simulink model "Simulink Model"  (R2020b)
settings: Solver=VariableStepAuto  StartTime=0.0  StopTime=10  RelTol=1e-3
undefined symbols (not defined in the file): a1, a2, g, R, r, v1, v2, v3, w, x, y, z
libraries: simulink_extras x1
settings Model: Creator=Dow69  LastModifiedBy=Dow69

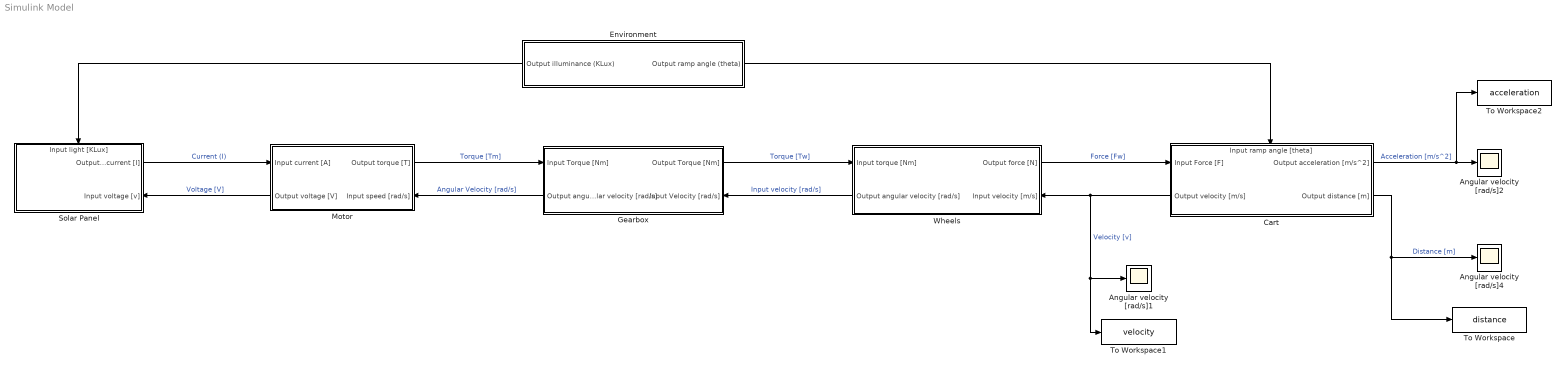
== system Simulink Model ==
  Angular velocity [rad/s]1 : Scope
  Angular velocity [rad/s]2 : Scope
  Angular velocity [rad/s]4 : Scope
  Cart : Subsystem  mask{m=1.319}
      mask prompts: m "Enter cart mass in kg"
      settings: PortSchema="{\"entries\":[{\"content\":{\"sides\":[{\"content\":{\"connectorIds\":[\"In1\",\"Out3\"]},\"type\":\"ConnectorPlacement.EquallySpacedRectSide\",\"uuid\":\"405a4784-f51f-4905-a480-0161a7144eef\"},{\"content\":{\"connectorIds\":[\"Out1\",\"Out2\"],\"side\":\"RIGHT\"},\"type\":\"ConnectorPlacement.EquallySpacedRectSide\",\"uuid\":\"ea7e0711-03fc-41b1-ba47-98d5601a56bc\"},{\"content\":{\"connectorIds\":[\"In2\"],\"side\":\"TOP\"},\"type\":\"ConnectorPlacement.EquallySpacedRectSide\",\"uuid\":\"329a5e39-ca06-4825-98ae-3bcb1db21222\"},{\"content\":{\"connectorIds\":[],\"side\":\"HIDDEN\"},\"type\":\"ConnectorPlacement.EquallySpacedRectSide\",\"uuid\":\"bdc78aba-688e-4dc2-92c3-421802cb88ce\"}]},\"type\":\"ConnectorPlacement.EquallySpacedConnector\",\"uuid\":\"ce64d1b9-0ca5-491b-8110-30a1d080445d\"}],\"packageUris\":[\"http://schema.mathworks.com/mf0/Connector/R2020b\"],\"version\":\"1.0\"}"
  Environment : Subsystem  mask{L=20, a=6.1}
      mask prompts: L "Enter illuminance in KLux"; a "Enter angle in degrees"
      settings: PortSchema="{\"entries\":[{\"content\":{\"sides\":[{\"content\":{\"connectorIds\":[\"Out2\"]},\"type\":\"ConnectorPlacement.EquallySpacedRectSide\",\"uuid\":\"216ba352-b268-472c-abbe-3cb1921569eb\"},{\"content\":{\"connectorIds\":[\"Out1\"],\"side\":\"RIGHT\"},\"type\":\"ConnectorPlacement.EquallySpacedRectSide\",\"uuid\":\"9aa5a236-758d-475f-983b-3b65685f354e\"},{\"content\":{\"connectorIds\":[],\"side\":\"TOP\"},\"type\":\"ConnectorPlacement.EquallySpacedRectSide\",\"uuid\":\"b54bcaaf-885b-4bc1-bf6d-84ce1f01bed9\"},{\"content\":{\"connectorIds\":[],\"side\":\"HIDDEN\"},\"type\":\"ConnectorPlacement.EquallySpacedRectSide\",\"uuid\":\"dd7d4bf7-52e6-41b8-b6d7-f11b8ad94410\"}]},\"type\":\"ConnectorPlacement.EquallySpacedConnector\",\"uuid\":\"024e2dd2-e0e3-4e08-8446-8a7f5dd20cd0\"}],\"packageUris\":[\"http://schema.mathworks.com/mf0/Connector/R2020b\"],\"version\":\"1.0\"}"
  Gearbox : Subsystem
      settings: PortSchema="{\"entries\":[{\"content\":{\"sides\":[{\"content\":{\"connectorIds\":[\"In1\",\"Out2\"]},\"type\":\"ConnectorPlacement.EquallySpacedRectSide\",\"uuid\":\"8709382a-be33-43d3-8815-e6eab9f7b0e2\"},{\"content\":{\"connectorIds\":[\"Out1\",\"In2\"],\"side\":\"RIGHT\"},\"type\":\"ConnectorPlacement.EquallySpacedRectSide\",\"uuid\":\"0ff964dc-029b-47ae-a4ba-260b3c732ea2\"},{\"content\":{\"connectorIds\":[],\"side\":\"TOP\"},\"type\":\"ConnectorPlacement.EquallySpacedRectSide\",\"uuid\":\"270be714-ac21-48e6-9a25-87552b992944\"},{\"content\":{\"connectorIds\":[],\"side\":\"HIDDEN\"},\"type\":\"ConnectorPlacement.EquallySpacedRectSide\",\"uuid\":\"9bfe0afb-4326-44a4-9bc7-f5e5f9747662\"}]},\"type\":\"ConnectorPlacement.EquallySpacedConnector\",\"uuid\":\"0c65735c-987a-4693-bab6-a5fdb23f2f10\"}],\"packageUris\":[\"http://schema.mathworks.com/mf0/Connector/R2020b\"],\"version\":\"1.0\"}"
  Motor : Subsystem
      settings: PortSchema="{\"entries\":[{\"content\":{\"sides\":[{\"content\":{\"connectorIds\":[\"In1\",\"Out2\"]},\"type\":\"ConnectorPlacement.EquallySpacedRectSide\",\"uuid\":\"8709382a-be33-43d3-8815-e6eab9f7b0e2\"},{\"content\":{\"connectorIds\":[\"Out1\",\"In2\"],\"side\":\"RIGHT\"},\"type\":\"ConnectorPlacement.EquallySpacedRectSide\",\"uuid\":\"0ff964dc-029b-47ae-a4ba-260b3c732ea2\"},{\"content\":{\"connectorIds\":[],\"side\":\"TOP\"},\"type\":\"ConnectorPlacement.EquallySpacedRectSide\",\"uuid\":\"270be714-ac21-48e6-9a25-87552b992944\"},{\"content\":{\"connectorIds\":[],\"side\":\"HIDDEN\"},\"type\":\"ConnectorPlacement.EquallySpacedRectSide\",\"uuid\":\"9bfe0afb-4326-44a4-9bc7-f5e5f9747662\"}]},\"type\":\"ConnectorPlacement.EquallySpacedConnector\",\"uuid\":\"0c65735c-987a-4693-bab6-a5fdb23f2f10\"}],\"packageUris\":[\"http://schema.mathworks.com/mf0/Connector/R2020b\"],\"version\":\"1.0\"}"
  Solar Panel : Subsystem
      settings: PortSchema="{\"entries\":[{\"content\":{\"sides\":[{\"content\":{\"connectorIds\":[]},\"type\":\"ConnectorPlacement.EquallySpacedRectSide\",\"uuid\":\"5e94bcc7-8ac1-4ecf-8100-02fdfcc2a02d\"},{\"content\":{\"connectorIds\":[\"Out1\",\"In2\"],\"side\":\"RIGHT\"},\"type\":\"ConnectorPlacement.EquallySpacedRectSide\",\"uuid\":\"50624a19-96d0-4675-bbd9-5831c6a2d3c8\"},{\"content\":{\"connectorIds\":[\"In1\"],\"side\":\"TOP\"},\"type\":\"ConnectorPlacement.EquallySpacedRectSide\",\"uuid\":\"7e0de8b2-f315-401a-bc17-e3e3ed5487a7\"},{\"content\":{\"connectorIds\":[],\"side\":\"HIDDEN\"},\"type\":\"ConnectorPlacement.EquallySpacedRectSide\",\"uuid\":\"ef6684b0-5930-4d11-963c-58087df45cf7\"}]},\"type\":\"ConnectorPlacement.EquallySpacedConnector\",\"uuid\":\"3a747598-d978-44ef-9553-272ae5ee0e87\"}],\"packageUris\":[\"http://schema.mathworks.com/mf0/Connector/R2020b\"],\"version\":\"1.0\"}"
  To Workspace : ToWorkspace  VariableName=distance  SaveFormat=Timeseries  SampleTime=-1
  To Workspace1 : ToWorkspace  VariableName=velocity  SaveFormat=Timeseries  SampleTime=-1
  To Workspace2 : ToWorkspace  VariableName=acceleration  SaveFormat=Timeseries  SampleTime=-1
  Wheels : Subsystem
      settings: PortSchema="{\"entries\":[{\"content\":{\"sides\":[{\"content\":{\"connectorIds\":[\"In1\",\"Out2\"]},\"type\":\"ConnectorPlacement.EquallySpacedRectSide\",\"uuid\":\"8709382a-be33-43d3-8815-e6eab9f7b0e2\"},{\"content\":{\"connectorIds\":[\"Out1\",\"In2\"],\"side\":\"RIGHT\"},\"type\":\"ConnectorPlacement.EquallySpacedRectSide\",\"uuid\":\"0ff964dc-029b-47ae-a4ba-260b3c732ea2\"},{\"content\":{\"connectorIds\":[],\"side\":\"TOP\"},\"type\":\"ConnectorPlacement.EquallySpacedRectSide\",\"uuid\":\"270be714-ac21-48e6-9a25-87552b992944\"},{\"content\":{\"connectorIds\":[],\"side\":\"HIDDEN\"},\"type\":\"ConnectorPlacement.EquallySpacedRectSide\",\"uuid\":\"9bfe0afb-4326-44a4-9bc7-f5e5f9747662\"}]},\"type\":\"ConnectorPlacement.EquallySpacedConnector\",\"uuid\":\"0c65735c-987a-4693-bab6-a5fdb23f2f10\"}],\"packageUris\":[\"http://schema.mathworks.com/mf0/Connector/R2020b\"],\"version\":\"1.0\"}"
  wires:
  Environment/1(Output illuminance (KLux)) -> Solar Panel/1(Input light [KLux])
  Motor/1(Output torque [T]) -> Gearbox/1(Input Torque [Nm])  "Torque [Tm]"
  Gearbox/1(Output Torque [Nm]) -> Wheels/1(Input torque [Nm])  "Torque [Tw]"
  Wheels/2(Output angular velocity [rad/s]) -> Gearbox/2(Input Velocity [rad/s])  "Input velocity [rad/s]"
  Wheels/1(Output force [N]) -> Cart/1(Input Force [F])  "Force [Fw]"
  Environment/2(Output ramp angle (theta)) -> Cart/2(Input ramp angle [theta])
  Cart/2(Output distance [m]) -> To Workspace/1, Angular velocity [rad/s]4/1  "Distance [m]"
  Gearbox/2(Output angular velocity [rad/s]) -> Motor/2(Input speed [rad/s])  "Angular Velocity [rad/s]"
  Cart/3(Output velocity [m/s]) -> To Workspace1/1, Angular velocity [rad/s]1/1, Wheels/2(Input velocity [m/s])  "Velocity [v]"
  Solar Panel/1(Output current [I]) -> Motor/1(Input current [A])  "Current (I)"
  Motor/2(Output voltage [V]) -> Solar Panel/2(Input voltage [v])  "Voltage [V]"
  Cart/1(Output acceleration [m/s^2]) -> Angular velocity [rad/s]2/1, To Workspace2/1  "Acceleration [m/s^2]"

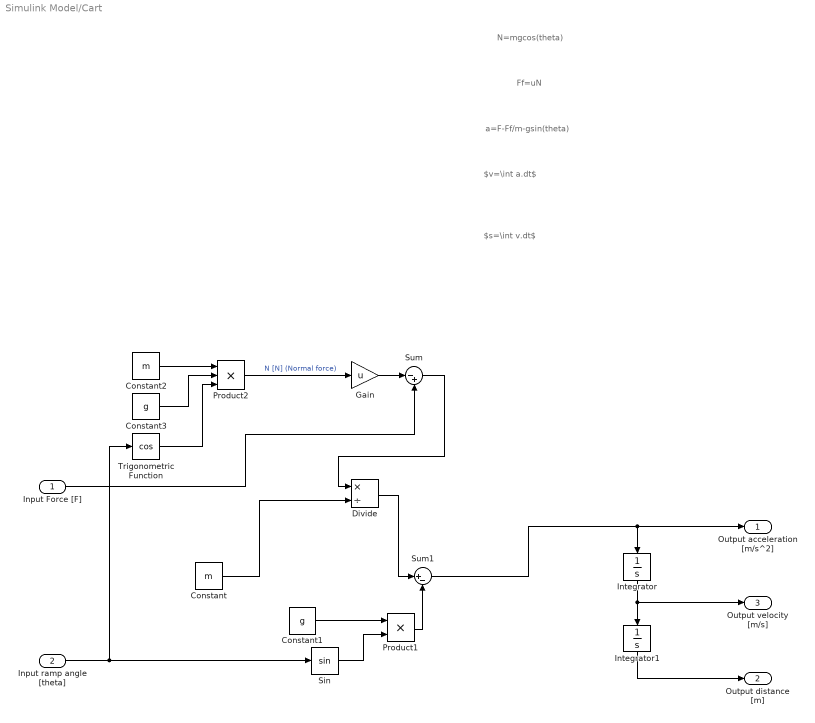
== system Simulink Model/Cart ==
  note: $s=\int v.dt$
  note: $v=\int a.dt$
  note: a=F-Ff/m-gsin(theta)
  note: Ff=uN
  note: N=mgcos(theta)
  Input Force [F] : Inport
  Input ramp angle [theta] : Inport  Port=2
  Constant : Constant  Value=m
  Constant1 : Constant  Value=g
  Constant2 : Constant  Value=m
  Constant3 : Constant  Value=g
  Divide : Product  Inputs=*/
  Gain : Gain  Gain=u
  Integrator : Integrator
  Integrator1 : Integrator
  Product1 : Product
  Product2 : Product  Inputs=3
  Sin : Trigonometry
  Sum : Sum  Inputs=|-+
  Sum1 : Sum  Inputs=|+-
  Trigonometric Function : Trigonometry  Operator=cos
  Output acceleration [m/s^2] : Outport
  Output distance [m] : Outport  Port=2
  Output velocity [m/s] : Outport  Port=3
  wires:
  Input ramp angle [theta]/1 -> Sin/1, Trigonometric Function/1
  Constant1/1 -> Product1/1
  Integrator/1 -> Output velocity [m/s]/1, Integrator1/1
  Integrator1/1 -> Output distance [m]/1
  Sin/1 -> Product1/2
  Trigonometric Function/1 -> Product2/3
  Constant3/1 -> Product2/2
  Constant2/1 -> Product2/1
  Product2/1 -> Gain/1  "N [N] (Normal force)"
  Product1/1 -> Sum1/2
  Constant/1 -> Divide/2
  Gain/1 -> Sum/1
  Input Force [F]/1 -> Sum/2
  Sum/1 -> Divide/1
  Divide/1 -> Sum1/1
  Sum1/1 -> Integrator/1, Output acceleration [m/s^2]/1

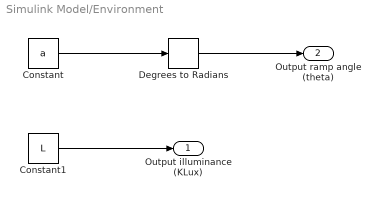
== system Simulink Model/Environment ==
  Constant : Constant  Value=a
  Constant1 : Constant  Value=L
  Degrees to Radians : simulink_extras/Transformations/Degrees to Radians
  Output illuminance (KLux) : Outport
  Output ramp angle (theta) : Outport  Port=2
  wires:
  Constant1/1 -> Output illuminance (KLux)/1
  Constant/1 -> Degrees to Radians/1
  Degrees to Radians/1 -> Output ramp angle (theta)/1

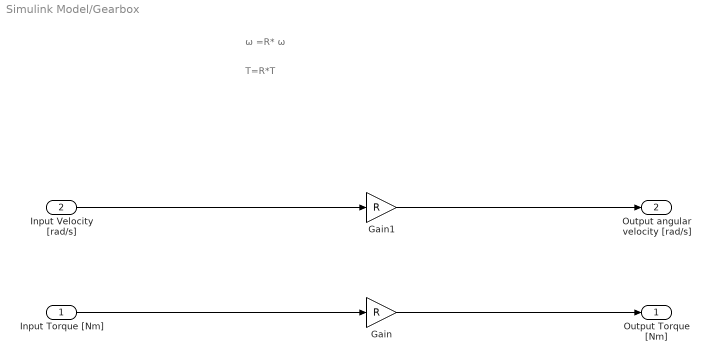
== system Simulink Model/Gearbox ==
  note: T=R*T
  note: ω =R* ω
  Input Torque [Nm] : Inport
  Input Velocity [rad/s] : Inport  Port=2
  Gain : Gain  Gain=R
  Gain1 : Gain  Gain=R
  Output Torque [Nm] : Outport
  Output angular velocity [rad/s] : Outport  Port=2
  wires:
  Input Velocity [rad/s]/1 -> Gain1/1
  Gain1/1 -> Output angular velocity [rad/s]/1
  Gain/1 -> Output Torque [Nm]/1
  Input Torque [Nm]/1 -> Gain/1

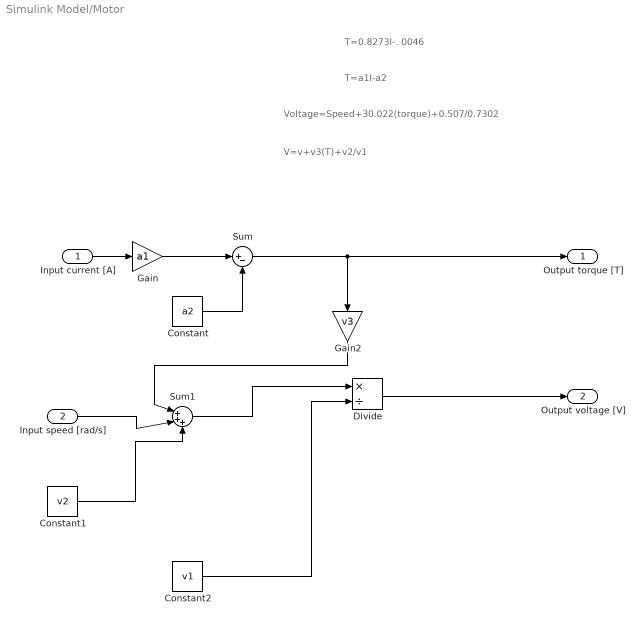
== system Simulink Model/Motor ==
  note: Voltage=Speed+30.022(torque)+0.507/0.7302
  note: T=0.8273I-. 0046
  note: V=v+v3(T)+v2/v1
  note: T=a1I-a2
  Input current [A] : Inport
  Input speed [rad/s] : Inport  Port=2
  Constant : Constant  Value=a2
  Constant1 : Constant  Value=v2
  Constant2 : Constant  Value=v1
  Divide : Product  Inputs=*/
  Gain : Gain  Gain=a1
  Gain2 : Gain  Gain=v3
  Sum : Sum  Inputs=|+-
  Sum1 : Sum  Inputs=|+++
  Output torque [T] : Outport
  Output voltage [V] : Outport  Port=2
  wires:
  Input current [A]/1 -> Gain/1
  Sum/1 -> Gain2/1, Output torque [T]/1
  Gain/1 -> Sum/1
  Constant/1 -> Sum/2
  Constant1/1 -> Sum1/3
  Constant2/1 -> Divide/2
  Input speed [rad/s]/1 -> Sum1/2
  Divide/1 -> Output voltage [V]/1
  Sum1/1 -> Divide/1
  Gain2/1 -> Sum1/1

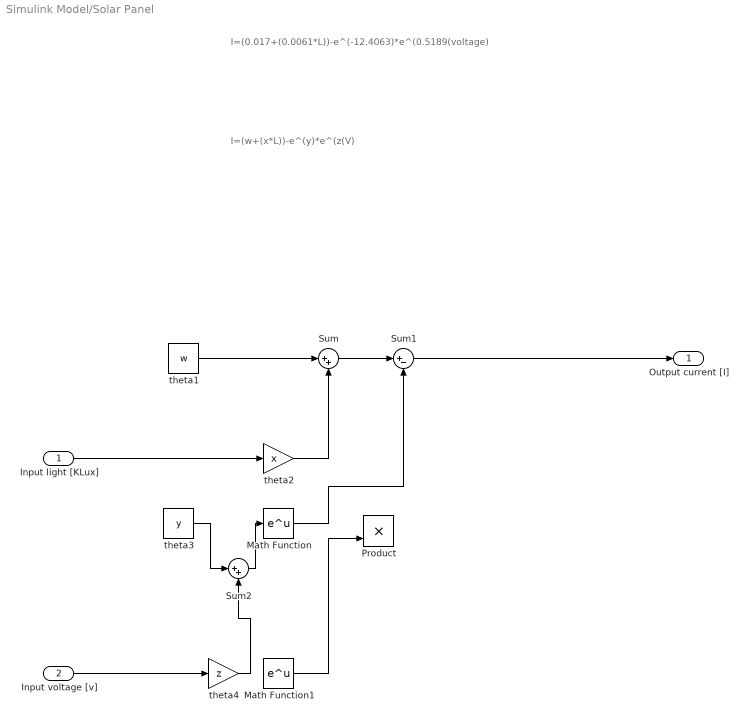
== system Simulink Model/Solar Panel ==
  note: I=(w+(x*L))-e^(y)*e^(z(V)
  note: I=(0.017+(0.0061*L))-e^(-12.4063)*e^(0.5189(voltage)
  Input light [KLux] : Inport
  Input voltage [v] : Inport  Port=2
  Math Function : Math  SaturateOnIntegerOverflow=on
  Math Function1 : Math  SaturateOnIntegerOverflow=on
  Product : Product
  Sum : Sum  Inputs=|++
  Sum1 : Sum  Inputs=|+-
  Sum2 : Sum  Inputs=|++
  theta1 : Constant  Value=w
  theta2 : Gain  Gain=x
  theta3 : Constant  Value=y
  theta4 : Gain  Gain=z
  Output current [I] : Outport
  wires:
  theta1/1 -> Sum/1
  Input light [KLux]/1 -> theta2/1
  theta2/1 -> Sum/2
  theta3/1 -> Sum2/1
  Math Function/1 -> Sum1/2
  Math Function1/1 -> Product/2
  Sum/1 -> Sum1/1
  Sum1/1 -> Output current [I]/1
  Input voltage [v]/1 -> theta4/1
  theta4/1 -> Sum2/2
  Sum2/1 -> Math Function/1

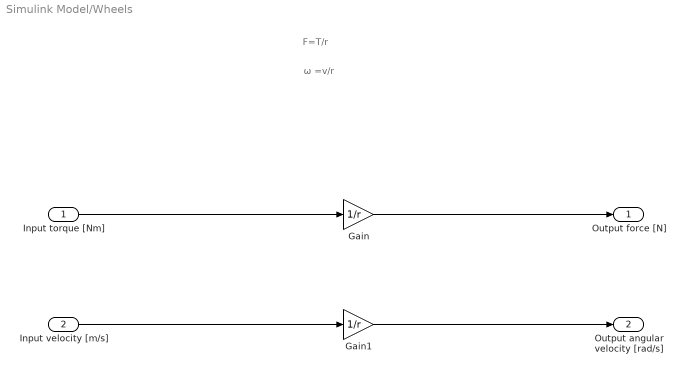
== system Simulink Model/Wheels ==
  note: ω =v/r
  note: F=T/r
  Input torque [Nm] : Inport
  Input velocity [m/s] : Inport  Port=2
  Gain : Gain  Gain=1/r
  Gain1 : Gain  Gain=1/r
  Output force [N] : Outport
  Output angular velocity [rad/s] : Outport  Port=2
  wires:
  Input torque [Nm]/1 -> Gain/1
  Input velocity [m/s]/1 -> Gain1/1
  Gain1/1 -> Output angular velocity [rad/s]/1
  Gain/1 -> Output force [N]/1
